simulink model "circuit1"  (R2017b)
settings: Solver=VariableStepAuto  StartTime=0.0  StopTime=10.0  MaxStep=1e-4  RelTol=1e-3
libraries: powerlib x12
settings Model: Creator=hansmariushagen  LastModifiedBy=hansmariushagen

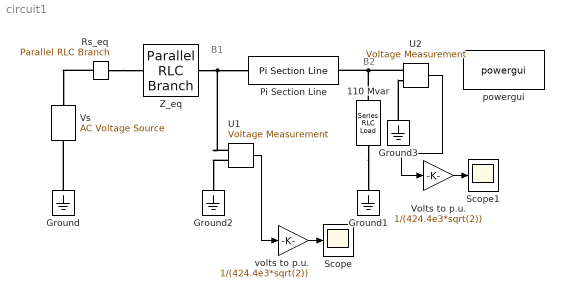
== system circuit1 ==
  note: B2
  note: B1
  110 Mvar : powerlib/Elements/Series RLC Load  LConnTagsString=a  RConnTagsString=__new0  NominalVoltage=424.4e3  NominalFrequency=60  ActivePower=110e6/300  InductivePower=110e6  CapacitivePower=0  Setx0=off  InitialVoltage=0  SetiL0=off  InitialCurrent=0  Measurements=None  LoadType=constant Z
  Ground{,1..3} (4 alike) : powerlib/Elements/Ground  LConnTagsString=a
  Pi Section Line : powerlib/Elements/Pi Section Line  LConnTagsString=__new0  RConnTagsString=__new0  Frequency=60  Resistance=0.011  Inductance=0.8674e-3  Capacitance=13.41e-9  Length=300  PiSections=1  Measurements=None
      settings: AttributesFormatString=\n  SourceProductName=Simscape Power Systems  SourceProductBaseCode=PS
  Rs_eq : powerlib/Elements/Parallel RLC Branch  LConnTagsString=a  RConnTagsString=__new0  BranchType=R  Resistance=2  Inductance=26.525e-3  SetiL0=off  InitialCurrent=0  Capacitance=117.84e-6  Setx0=off  InitialVoltage=0  Measurements=None
  Scope : Scope
  Scope1 : Scope
  U1 : powerlib/Measurements/Voltage Measurement  PhasorSimulation=off  OutputType=Complex  PSBequivalent=0
  U2 : powerlib/Measurements/Voltage Measurement  PhasorSimulation=off  OutputType=Complex  PSBequivalent=0
  Volts to p.u. : Gain  Gain=1/(424.4e3*sqrt(2))
  Vs : powerlib/Electrical Sources/AC Voltage Source  Amplitude=424.4e3*sqrt(2)  Phase=0  Frequency=0.60  SampleTime=0  Measurements=None  BusType=swing  Pref=10e3  Qref=0  Qmin=-inf  Qmax=+inf
  Z_eq : powerlib/Elements/Parallel RLC Branch  LConnTagsString=a  RConnTagsString=__new0  BranchType=RLC  Resistance=180.1  Inductance=26.525e-3  SetiL0=off  InitialCurrent=0  Capacitance=117.84e-6  Setx0=off  InitialVoltage=0  Measurements=None
  powergui : powerlib/powergui  Priority=1  SimulationMode=Continuous  SampleTime=50e-6  frequency=60  Iterations=50  frequencyindice=0.6  Pbase=100e6  ErrMax=1e-4  UnitsV=kV  UnitsW=MW  buscounter=0  FunctionMessages=off  echomessages=off  EnableUseOfTLC=off  CurrentSourceSwitches=off  DisableSnubberDevices=off  DisableRonSwitches=off  DisableVfSwitches=off  DisplayEquations=off  SolverType=Tustin/Backward Euler (TBE)  Interpol=off  ExternalGateDelay=off  methode=off  Ts=100  x0status=blocks  SPID=on  SwTol=0  HookPort=off  RestoreLinks=warning  ResistiveCurrentMeasurement=off  Frange=[0:2:500]  Ylog=off  Xlog=on  ShowGrid=off  save=off  variable=ZData  structure=0  ZoomFFT=off  StartTime=0.0  cycles=1  DisplayStyle=1  fundamental=60  FreqAxis=off  MaxFrequency=1000  frequencyindicesteady=1  RmsSteady=1  display=off
  volts to p.u. : Gain  Gain=1/(424.4e3*sqrt(2))
  wires:
  U1/1 -> volts to p.u./1
  volts to p.u./1 -> Scope/1
  Volts to p.u./1 -> Scope1/1
  U2/1 -> Volts to p.u./1
  connections:
  Rs_eq/LConn1 -- Vs/RConn1
  Rs_eq/RConn1 -- Z_eq/LConn1
  Z_eq/RConn1 -- U1/LConn1 -- Pi Section Line/LConn1
  110 Mvar/LConn1 -- Pi Section Line/RConn1 -- U2/LConn1
  110 Mvar/RConn1 -- Ground1/LConn1
  Ground/LConn1 -- Vs/LConn1
  U1/LConn2 -- Ground2/LConn1
  Ground3/LConn1 -- U2/LConn2
